simulink model "w"  (Simulink 8.6)
settings: Solver=VariableStepAuto  StartTime=0.0  StopTime=t_end  MaxStep=h_max  RelTol=1e-3
InitFcn:
  | w_h_init
StopFcn:
  | w_stop
values from neighbouring files (symbols this model uses):
  a1 = 1    [w_h_init.m]
  a2 = 3    [w_h_init.m]
  k1 = 1.5    [w_h_init.m]
  k2 = 2    [w_h_init.m]
  t_end = 4    [w_h_init.m]
settings Model: Creator=etsu-laptop  LastModifiedBy=etsu-laptop
settings DataIOCC: SaveFormat=Dataset  SignalLoggingSaveFormat=Dataset
settings OptimizationCC: ExpressionDepthLimit=128
settings DebuggingCC: UnderspecifiedInitializationDetection=Simplified  MergeDetectMultiDrivingBlocksExec=error  SolverPrmCheckMsg=none  FcnCallInpInsideContextMsg=EnableAllAsError  StateNameClashWarn=none
settings HardwareCC: ProdBitPerPointer=64  ProdLargestAtomicFloat=Float  ProdIntDivRoundTo=Zero  ProdEndianess=LittleEndian  ProdWordSize=64  ProdHWDeviceType=Intel->x86-64 (Windows64)
settings GRTTargetCC: GeneratePreprocessorConditionals=Use local settings  CombineOutputUpdateFcns=on  GRTInterface=off
settings ConfigComp: CovModelRefEnable=off

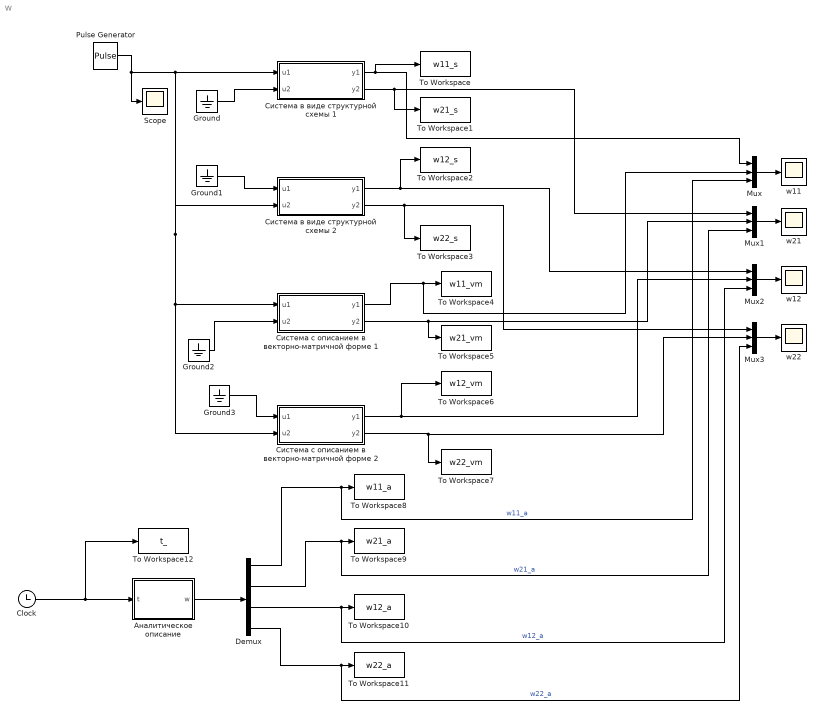
== system w ==
  Clock : Clock
  Demux : Demux
  Ground{,1..3} (4 alike) : Ground
  Mux{,1..3} (4 alike) : Mux  Inputs=3
  Pulse Generator : DiscretePulseGenerator  PulseType=Time based  Amplitude=1/(0.001*1.1*t_end)  Period=1.1*t_end  PulseWidth=0.1
  Scope : Scope
  To Workspace : ToWorkspace  VariableName=w11_s  SampleTime=-1
  To Workspace1 : ToWorkspace  VariableName=w21_s  SampleTime=-1
  To Workspace10 : ToWorkspace  VariableName=w12_a  SampleTime=-1
  To Workspace11 : ToWorkspace  VariableName=w22_a  SampleTime=-1
  To Workspace12 : ToWorkspace  VariableName=t_  SampleTime=-1
  To Workspace2 : ToWorkspace  VariableName=w12_s  SampleTime=-1
  To Workspace3 : ToWorkspace  VariableName=w22_s  SampleTime=-1
  To Workspace4 : ToWorkspace  VariableName=w11_vm  SampleTime=-1
  To Workspace5 : ToWorkspace  VariableName=w21_vm  SampleTime=-1
  To Workspace6 : ToWorkspace  VariableName=w12_vm  SampleTime=-1
  To Workspace7 : ToWorkspace  VariableName=w22_vm  SampleTime=-1
  To Workspace8 : ToWorkspace  VariableName=w11_a  SampleTime=-1
  To Workspace9 : ToWorkspace  VariableName=w21_a  SampleTime=-1
  w{11..12,21..22} (4 alike) : Scope
  Аналитическое описание : MATLAB Function  TreatAsAtomicUnit=on
  Система в виде структурной схемы 1 : Subsystem
  Система в виде структурной схемы 2 : Subsystem
  Система с описанием в векторно-матричной форме 1 : Subsystem
  Система с описанием в векторно-матричной форме 2 : Subsystem
  wires:
  Ground/1 -> Система в виде структурной схемы 1/2(u2)
  Ground1/1 -> Система в виде структурной схемы 2/1(u1)
  Mux/1 -> w11/1
  Система в виде структурной схемы 1/1(y1) -> To Workspace/1, Mux/1
  Система в виде структурной схемы 1/2(y2) -> To Workspace1/1, Mux1/1
  Mux1/1 -> w21/1
  Mux2/1 -> w12/1
  Mux3/1 -> w22/1
  Система в виде структурной схемы 2/2(y2) -> Mux3/1, To Workspace3/1
  Система в виде структурной схемы 2/1(y1) -> To Workspace2/1, Mux2/1
  Система с описанием в векторно-матричной форме 1/2(y2) -> Mux1/2, To Workspace5/1
  Система с описанием в векторно-матричной форме 1/1(y1) -> Mux/2, To Workspace4/1
  Система с описанием в векторно-матричной форме 2/2(y2) -> Mux3/2, To Workspace7/1
  Система с описанием в векторно-матричной форме 2/1(y1) -> Mux2/2, To Workspace6/1
  Ground2/1 -> Система с описанием в векторно-матричной форме 1/2(u2)
  Pulse Generator/1 -> Система с описанием в векторно-матричной форме 2/2(u2), Система с описанием в векторно-матричной форме 1/1(u1), Система в виде структурной схемы 2/2(u2), Система в виде структурной схемы 1/1(u1), Scope/1
  Ground3/1 -> Система с описанием в векторно-матричной форме 2/1(u1)
  Clock/1 -> Аналитическое описание/1(t), To Workspace12/1
  Аналитическое описание/1(w) -> Demux/1
  Demux/1 -> Mux/3, To Workspace8/1  "w11_a"
  Demux/2 -> Mux1/3, To Workspace9/1  "w21_a"
  Demux/3 -> Mux2/3, To Workspace10/1  "w12_a"
  Demux/4 -> Mux3/3, To Workspace11/1  "w22_a"

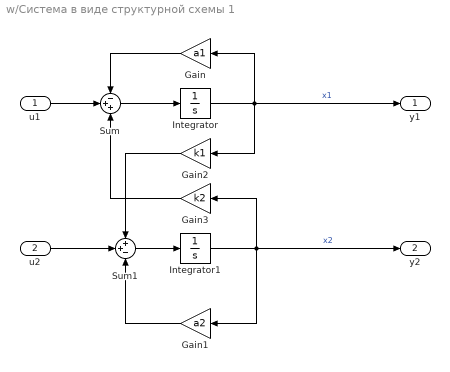
== system w/Система в виде структурной схемы 1 ==
  u1 : Inport
  u2 : Inport  Port=2
  Gain : Gain  Gain=a1
  Gain1 : Gain  Gain=a2
  Gain2 : Gain  Gain=k1
  Gain3 : Gain  Gain=k2
  Integrator : Integrator
  Integrator1 : Integrator
  Sum : Sum  Inputs=-++
  Sum1 : Sum  Inputs=++-
  y1 : Outport
  y2 : Outport  Port=2
  wires:
  u1/1 -> Sum/2
  u2/1 -> Sum1/2
  Sum/1 -> Integrator/1
  Sum1/1 -> Integrator1/1
  Integrator/1 -> Gain/1, Gain2/1, y1/1  "x1"
  Integrator1/1 -> Gain1/1, Gain3/1, y2/1  "x2"
  Gain/1 -> Sum/1
  Gain1/1 -> Sum1/3
  Gain3/1 -> Sum/3
  Gain2/1 -> Sum1/1

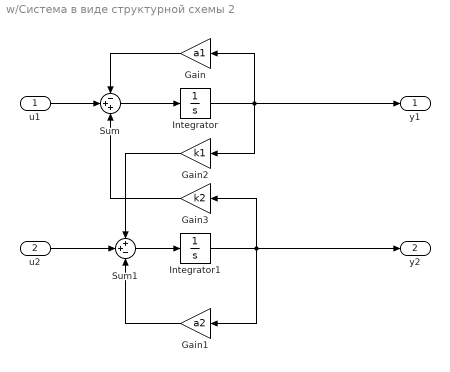
== system w/Система в виде структурной схемы 2 ==
  u1 : Inport
  u2 : Inport  Port=2
  Gain : Gain  Gain=a1
  Gain1 : Gain  Gain=a2
  Gain2 : Gain  Gain=k1
  Gain3 : Gain  Gain=k2
  Integrator : Integrator
  Integrator1 : Integrator
  Sum : Sum  Inputs=-++
  Sum1 : Sum  Inputs=++-
  y1 : Outport
  y2 : Outport  Port=2
  wires:
  Gain2/1 -> Sum1/1
  Gain3/1 -> Sum/3
  Gain1/1 -> Sum1/3
  Gain/1 -> Sum/1
  Integrator1/1 -> y2/1, Gain3/1, Gain1/1
  Integrator/1 -> y1/1, Gain2/1, Gain/1
  Sum1/1 -> Integrator1/1
  Sum/1 -> Integrator/1
  u2/1 -> Sum1/2
  u1/1 -> Sum/2

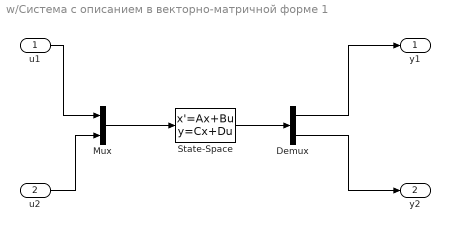
== system w/Система с описанием в векторно-матричной форме 1 ==
  u1 : Inport
  u2 : Inport  Port=2
  Demux : Demux  Outputs=2
  Mux : Mux  Inputs=2
  State-Space : StateSpace  A=[-a1 k2; k1 -a2]  B=eye(2)  C=eye(2)  D=zeros(2)  X0=0
  y1 : Outport
  y2 : Outport  Port=2
  wires:
  u2/1 -> Mux/2
  u1/1 -> Mux/1
  Mux/1 -> State-Space/1
  State-Space/1 -> Demux/1
  Demux/1 -> y1/1
  Demux/2 -> y2/1

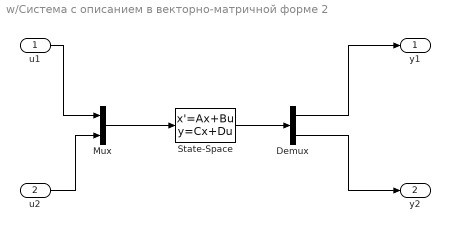
== system w/Система с описанием в векторно-матричной форме 2 ==
  u1 : Inport
  u2 : Inport  Port=2
  Demux : Demux  Outputs=2
  Mux : Mux  Inputs=2
  State-Space : StateSpace  A=[-a1 k2; k1 -a2]  B=eye(2)  C=eye(2)  D=zeros(2)  X0=0
  y1 : Outport
  y2 : Outport  Port=2
  wires:
  Demux/2 -> y2/1
  Demux/1 -> y1/1
  State-Space/1 -> Demux/1
  Mux/1 -> State-Space/1
  u1/1 -> Mux/1
  u2/1 -> Mux/2

== matlab function Аналитическое описание ==
  data: t input double; w output double
function w = fcn(t)
M1=1/8*[6 4; 3 2];
M2=1/8*[2 -4; -3 6];
l1=0;
l2=-4;
w_=M1*exp(l1*t)+M2*exp(l2*t);
w=reshape(w_,4,1);
